simulink model "matlab_model"  (R2023a)
settings: Solver=VariableStepAuto  StartTime=0.0  StopTime=40  RelTol=1e-3
values from neighbouring files (symbols this model uses):
  contact =     [param_cina_pitch.mat]    (also in param_cina_roll.mat; param_cina_yaw.mat; verifikasi_simulasi.mat)
  control =     [param_cina_pitch.mat]    (also in param_cina_roll.mat; param_cina_yaw.mat; verifikasi_simulasi.mat)
  D = 0    [23_3_24.mat]    (also in latihanMPC.m; modelYawSpeed.mat; mpc1.mat; nonLinear.m)
  dragCoeffMov = 0.01    [23_3_24.mat]    (also in mpcDoang.mat; param_cina_pitch.mat; param_cina_roll.mat; param_cina_yaw.mat)
  dx = [dx1;dx2;dx3;dx4;dx5;dx6]    [nonLinear.m]
  g = 9.81    [param_cina_pitch.mat]    (also in param_cina_roll.mat; param_cina_yaw.mat; verifikasi_simulasi.mat)
  mass = 0.8    [nonLinear.m]    (also in param_cina_pitch.mat = 1.371; param_cina_roll.mat = 1.371; param_cina_yaw.mat = 1.371; verifikasi_simulasi.mat = 1.371)
  ModelParam_rotorCm = 8e-08    [param_cina_pitch.mat]    (also in param_cina_roll.mat; param_cina_yaw.mat)
  ModelParam_rotorCt = 4.27e-06    [param_cina_pitch.mat]    (also in param_cina_roll.mat; param_cina_yaw.mat)
  ModelParam_uavR = 0.225    [param_cina_pitch.mat]    (also in param_cina_roll.mat; param_cina_yaw.mat)
  p = angRate.Data(:,1)    [log_analisis.m]
  pitch = ATT(:,6)    [log_analisis.m]    (also in param_cina_pitch.mat = [0 0 0 0 0 0 0 0 0 0 0 0 ... (161 elements, 161x1)]; param_cina_roll.mat = [0 0 0 0 0 0 0 0 0 0 0 0 ... (161 elements, 161x1)]; param_cina_yaw.mat = [0 0 0 0 0 0 0 0 0 0 0 0 ... (161 elements, 161x1)]; verifikasi_simulasi.mat = [0 0 0 0 0 0 0 0 0 0 0 0 ... (161 elements, 161x1)])
  q = angRate.Data(:,2)    [log_analisis.m]
  r = [0 0 0 ... (first row only)    [latihanMPC.m]    (also in log_analisis.m = angRate.Data(:,3))
  ref_height = 488    [param_cina_pitch.mat]    (also in param_cina_roll.mat; param_cina_yaw.mat; verifikasi_simulasi.mat)
  ref_lat = 47.397742    [param_cina_pitch.mat]    (also in param_cina_roll.mat; param_cina_yaw.mat; verifikasi_simulasi.mat)
  ref_lon = 8.545594    [param_cina_pitch.mat]    (also in param_cina_roll.mat; param_cina_yaw.mat; verifikasi_simulasi.mat)
  roll = ATT(:,4)    [log_analisis.m]    (also in param_cina_pitch.mat = [0 0 0 0 0 0 0 0 0 0 0 0 ... (161 elements, 161x1)]; param_cina_roll.mat = [0 0 0 0 0 0 0 0 0 0 0 0 ... (161 elements, 161x1)]; param_cina_yaw.mat = [0 0 0 0 0 0 0 0 0 0 0 0 ... (161 elements, 161x1)]; verifikasi_simulasi.mat = [0 0 0 0 0 0 0 0 0 0 0 0 ... (161 elements, 161x1)])
  rotorDir = [-1 -1 1 1]    [param_cina_pitch.mat]    (also in param_cina_roll.mat; param_cina_yaw.mat; verifikasi_simulasi.mat)
  rotorPositions = [0.1815  -0.1815  0.1815  -0.1815; 0.1815  -0.1815  -0.1815  0.1815; 0  0  0  0]    [param_cina_pitch.mat]    (also in param_cina_roll.mat; param_cina_yaw.mat; verifikasi_simulasi.mat)
  rotorThrustMax = 2    [param_cina_pitch.mat]    (also in param_cina_roll.mat = 3.5; param_cina_yaw.mat = 4; verifikasi_simulasi.mat = 1.83)
  rotorTimeConst = 0.005    [param_cina_pitch.mat]    (also in param_cina_roll.mat; param_cina_yaw.mat; verifikasi_simulasi.mat)
  rotorTorqueMax = 0.06    [param_cina_pitch.mat]    (also in param_cina_roll.mat; param_cina_yaw.mat; verifikasi_simulasi.mat)
  windVel = [0 0 0]    [param_cina_pitch.mat]    (also in param_cina_roll.mat; param_cina_yaw.mat; verifikasi_simulasi.mat)
  yaw = ATT(:,8)    [log_analisis.m]    (also in param_cina_pitch.mat = [0 0 0 0 0 0 0 0 0 0 0 0 ... (161 elements, 161x1)]; param_cina_roll.mat = [0 0 0 0 0 0 0 0 0 0 0 0 ... (161 elements, 161x1)]; param_cina_yaw.mat = [0 0 0 0 0 0 0 0 0 0 0 0 ... (161 elements, 161x1)]; verifikasi_simulasi.mat = [0 0 0 0 0 0 0 0 0 0 0 0 ... (161 elements, 161x1)])
undefined symbols (not defined in the file or in its folder): ddx, ddy, ddz, dy, dz, X, Y, Z
libraries: shared6dof x1, robotcorelib x1, simulink x1, sensorgpslib x1, mspsensorlib x1
settings Model: Creator=LENOVO  LastModifiedBy=LENOVO

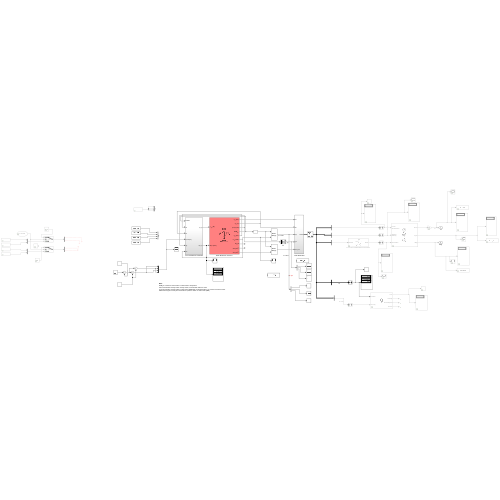
[thumbnail: Simulink's stored preview of the top-level diagram]
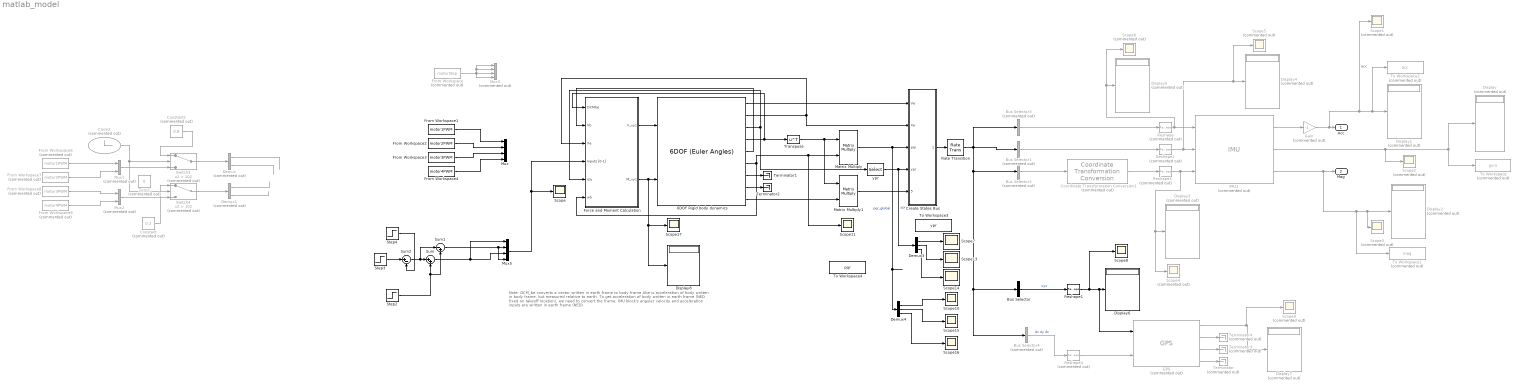
== system matlab_model ==
  note: Note:
      | DCM_be converts a vector written in earth frame to body frame
      | Abe is acceleration of body written in body frame, but measured relative to earth.
      | To get acceleration of body written in earth frame (NED fixed on takeoff location), we need to convert the frame.
      | IMU block's angular velocity and acceleration inputs are written in earth frame (NED)
  "6DOF Rigid body dynamics " : shared6dof/6DOF (Euler Angles)  units=Metric (MKS)  mtype=Fixed  rep=Quaternion  xme_0=[0,0,0]  Vm_0=init.vb  eul_0=[0;0;0]  pm_0=init.angRates  mass_0=mass  mass_e=0.5  mass_f=2.0  inertia=inertia  inertia_e=eye(3)  inertia_f=2*eye(3)  k_quat=1  vre_flag=on  abi_flag=on  aMode=aMode  xme_statename=''  Vm_statename=''  eul_statename=''  quat_statename=''  pm_statename=''  mass_statename=''
  Bus Selector : BusSelector  OutputSignals=X,Y,Z  OutputAsBus=on
  Bus Selector1 : BusSelector  Commented=on  OutputSignals=p,q,r  OutputAsBus=on
  Bus Selector2 : BusSelector  Commented=on  OutputSignals=yaw,pitch,roll  OutputAsBus=on
  Bus Selector3 : BusSelector  Commented=on  OutputSignals=ddx,ddy,ddz  OutputAsBus=on
  Bus Selector4 : BusSelector  Commented=on  OutputSignals=dx,dy,dz  OutputAsBus=on
  Clock2 : Clock  Commented=on
  Constant : Constant  Commented=on  Value=0.2
  Constant1 : Constant  Commented=on  Value=0.8
  Coordinate Transformation Conversion1 : robotcorelib/Coordinate Transformation Conversion  Commented=on  InputRepresentation=Euler Angles  InputEulerSequence=ZYX  ShowTrVecInputPort=on  OutputRepresentation=Quaternion  OutputEulerSequence=ZYX  ShowTrVecOutputPort=on  SimulateUsing=Interpreted execution
  Create States Bus : Subsystem
  Demux : Demux  Commented=on  Outputs=2
  Demux1 : Demux  Commented=on  Outputs=2
  Demux3 : Demux  Outputs=3
  Demux4 : Demux  Outputs=3
  Display{,1..5,7} (7 alike) : Display  Commented=on
  Display6 : Display
  Display8 : Display
  Force and Moment Calculation : Subsystem
  From Workspace : FromWorkspace  Commented=on  VariableName=motorStep
  From Workspace1 : FromWorkspace  VariableName=motor1PWM  SampleTime=0.25
  From Workspace2 : FromWorkspace  VariableName=motor2PWM  SampleTime=0.25
  From Workspace3 : FromWorkspace  VariableName=motor3PWM  SampleTime=0.25
  From Workspace4 : FromWorkspace  VariableName=motor4PWM  SampleTime=0.25
  From Workspace6 : FromWorkspace  Commented=on  VariableName=motor1PWM  SampleTime=0.01
  From Workspace7 : FromWorkspace  Commented=on  VariableName=motor2PWM  SampleTime=0.01
  From Workspace8 : FromWorkspace  Commented=on  VariableName=motor3PWM  SampleTime=0.01
  From Workspace9 : FromWorkspace  Commented=on  VariableName=motor4PWM  SampleTime=0.01
  GPS : sensorgpslib/GPS  Commented=on  DispRefFrame=NED  PositionInputFormat=Local  ReferenceLocation=[ref_lat ref_lon ref_height]  HorizontalPositionAccuracy=0.01  VerticalPositionAccuracy=0.01  VelocityAccuracy=0.01  DecayFactor=0.99  SeedDouble=67  SimulateUsing=Interpreted execution
      settings: LibrarySourceBlock=mspsensorlib/GPS
  Gain : Gain  Commented=on  Gain=-1
  IMU1 : mspsensorlib/IMU  Commented=on  DispRefFrame=NED  Temperature=25  MagneticFieldNED=[21.5 1.16 43.1]  MagneticFieldENU=[ -2.4169, 27.5550, 16.0849 ]  SeedDouble=87254  SimulateUsing=Interpreted execution  AccelParamsMeasurementRange=Inf  AccelParamsResolution=0  AccelParamsConstantBias=[ 0, 0, 0 ]  AccelParamsAxesMisalignment=[ 0, 0, 0 ]  AccelParamsNoiseDensity=0.0003  AccelParamsBiasInstability=[ 0, 0, 0 ]  AccelParamsRandomWalk=[ 0, 0, 0 ]  AccelParamsTemperatureBias=[ 0, 0, 0 ]  AccelParamsTemperatureScaleFactor=[ 0, 0, 0 ]  GyroParamsMeasurementRange=Inf  GyroParamsResolution=0  GyroParamsConstantBias=[ 0, 0, 0 ]  GyroParamsAxesMisalignment=[ 0, 0, 0 ]  GyroParamsAccelerationBias=0.0001  GyroParamsNoiseDensity=0.01  GyroParamsBiasInstability=[ 0, 0, 0 ]  GyroParamsRandomWalk=[ 0, 0, 0 ]  GyroParamsTemperatureBias=[ 0, 0, 0 ]  GyroParamsTemperatureScaleFactor=[ 0, 0, 0 ]  MagParamsMeasurementRange=Inf  MagParamsResolution=0  MagParamsConstantBias=[ 0, 0, 0 ]  MagParamsAxesMisalignment=[ 0, 0, 0 ]  MagParamsNoiseDensity=0.0005  MagParamsBiasInstability=[ 0, 0, 0 ]  MagParamsRandomWalk=[ 0, 0, 0 ]  MagParamsTemperatureBias=[ 0, 0, 0 ]  MagParamsTemperatureScaleFactor=[ 0, 0, 0 ]
  Matrix Multiply : Product  Multiplication=Matrix(*)
  Matrix Multiply1 : Product  Multiplication=Matrix(*)
  Mux : Mux
  Mux1 : Mux  Commented=on  Inputs=2
  Mux2 : Mux  Commented=on  Inputs=2
  Mux3 : Mux  Commented=on
  Mux5 : Mux
  Rate Transition : RateTransition  OutPortSampleTime=0.01
  Reshape{,2..4} (4 alike) : Reshape  Commented=on  OutputDimensionality=Row vector (2-D)
  Reshape1 : Reshape  OutputDimensionality=Row vector (2-D)
  Scope{,7..8,10..11,13..17} (10 alike) : Scope
  Scope{1..6,9} (7 alike) : Scope  Commented=on
  Step2 : Step  Time=0  After=0.9  SampleTime=0.25
  Step3 : Step  Time=10  After=0.01  SampleTime=0.25
  Step4 : Step  Time=11  After=0.01  SampleTime=0.25
  Sum : Sum  Inputs=|++
  Sum1 : Sum  Inputs=|-+
  Sum2 : Sum  Inputs=|+-
  Switch3 : Switch  Commented=on  Criteria=u2 > Threshold  Threshold=102  SaturateOnIntegerOverflow=off  InputSameDT=off
  Switch4 : Switch  Commented=on  Criteria=u2 > Threshold  Threshold=102  SaturateOnIntegerOverflow=off  InputSameDT=off
  Terminator : Terminator  Commented=on
  Terminator1 : Terminator
  Terminator2 : Terminator
  Terminator3 : Terminator  Commented=on
  Terminator4 : Terminator  Commented=on
  To Workspace : ToWorkspace  Commented=on  VariableName=gyro  SaveFormat=Timeseries  SampleTime=0.25
  To Workspace1 : ToWorkspace  Commented=on  VariableName=mag  SaveFormat=Timeseries  SampleTime=0.25
  To Workspace2 : ToWorkspace  Commented=on  VariableName=acc  SaveFormat=Timeseries  SampleTime=0.25
  To Workspace3 : ToWorkspace  VariableName=ypr  SaveFormat=Timeseries  SampleTime=0.25
  To Workspace4 : ToWorkspace  VariableName=pqr  SaveFormat=Timeseries  SampleTime=0.25
  Transpose : Math  Operator=transpose
  Zero1 : Constant  Commented=on  Value=0  OutDataTypeStr=Inherit: Inherit via back propagation
  ypr : Selector  InputPortWidth=3  IndexOptions=Index vector (dialog)  Indices=[3 2 1]  OutputSizes=1
  Acc : Outport
  Mag : Outport  Port=2
  wires:
  Force and Moment Calculation/2(M_xyz) -> Display8/1, Scope17/1, "6DOF Rigid body dynamics "/2
  Matrix Multiply/1 -> Demux4/1, Create States Bus/3(pqr)  "pqr_global"
  "6DOF Rigid body dynamics "/4 -> Force and Moment Calculation/1(DCMbe), Transpose/1
  "6DOF Rigid body dynamics "/3 -> Force and Moment Calculation/5(rpy), ypr/1
  "6DOF Rigid body dynamics "/5 -> Force and Moment Calculation/2(Vb)
  "6DOF Rigid body dynamics "/8 -> Terminator2/1
  "6DOF Rigid body dynamics "/7 -> Terminator1/1
  Transpose/1 -> Matrix Multiply1/1, Matrix Multiply/1
  ypr/1 -> Demux3/1, Create States Bus/4(ypr)  "ypr"
  "6DOF Rigid body dynamics "/9 -> Matrix Multiply1/2
  Force and Moment Calculation/1(F_xyz) -> "6DOF Rigid body dynamics "/1
  "6DOF Rigid body dynamics "/6 -> Scope11/1, Matrix Multiply/2, Force and Moment Calculation/6(wb)
  "6DOF Rigid body dynamics "/2 -> Create States Bus/2(Xe), Force and Moment Calculation/3(Xe)
  IMU1/2 -> Scope2/1, To Workspace/1, Display/1
  Gain/1 -> Scope1/1, To Workspace2/1, Display1/1, Acc/1  "acc"
  Reshape2/1 -> Scope5/1, Display4/1, IMU1/2
  Bus Selector2/1 -> Coordinate Transformation Conversion1/1
  Coordinate Transformation Conversion1/1 -> Reshape3/1
  Bus Selector1/1 -> Reshape2/1
  IMU1/3 -> To Workspace1/1, Scope3/1, Display2/1, Mag/1
  IMU1/1 -> Gain/1
  Bus Selector3/1 -> Reshape/1
  Reshape3/1 -> Scope4/1, Display3/1, IMU1/3
  "6DOF Rigid body dynamics "/1 -> Create States Bus/1(Ve)
  Matrix Multiply1/1 -> Create States Bus/5(acc_lnav)
  Create States Bus/1(States) -> Rate Transition/1
  Reshape/1 -> Scope6/1, Display5/1, IMU1/1
  Rate Transition/1 -> Bus Selector2/1, Bus Selector/1, Bus Selector4/1, Bus Selector1/1, Bus Selector3/1
  Bus Selector/1 -> Reshape1/1  "xyz"
  From Workspace6/1 -> Mux1/1
  From Workspace7/1 -> Mux1/2
  From Workspace8/1 -> Mux2/1
  From Workspace9/1 -> Mux2/2
  Mux1/1 -> Switch3/3
  Clock2/1 -> Switch4/2, Switch3/2
  Mux2/1 -> Switch4/3
  Switch3/1 -> Demux/1
  Switch4/1 -> Demux1/1
  Demux1/1 -> ?
  Demux1/2 -> ?
  Demux/1 -> ?
  Demux/2 -> ?
  Reshape1/1 -> Scope8/1, GPS/1, Display6/1
  Bus Selector4/1 -> Reshape4/1  "dx dy dz"
  Reshape4/1 -> GPS/2
  GPS/4 -> Terminator/1
  GPS/3 -> Terminator3/1
  GPS/2 -> Terminator4/1
  GPS/1 -> Scope9/1, Display7/1
  Constant/1 -> Switch4/1
  Constant1/1 -> Switch3/1
  From Workspace1/1 -> Mux/1
  From Workspace2/1 -> Mux/2
  From Workspace3/1 -> Mux/3
  From Workspace4/1 -> Mux/4
  From Workspace/1 -> Mux3/1, Mux3/2, Mux3/4, Mux3/3
  Demux3/2 -> Scope13/1
  Demux3/3 -> Scope14/1
  Demux3/1 -> Scope7/1
  Demux4/1 -> Scope10/1
  Demux4/2 -> Scope15/1
  Demux4/3 -> Scope16/1
  Step3/1 -> Sum2/1
  Sum1/1 -> Mux5/4, Mux5/2
  Step2/1 -> Sum1/2, Sum/2
  Sum2/1 -> Sum1/1, Sum/1
  Sum/1 -> Mux5/1, Mux5/3
  Step4/1 -> Sum2/2
  Mux5/1 -> Force and Moment Calculation/4(Inputs [0-1]), Scope/1

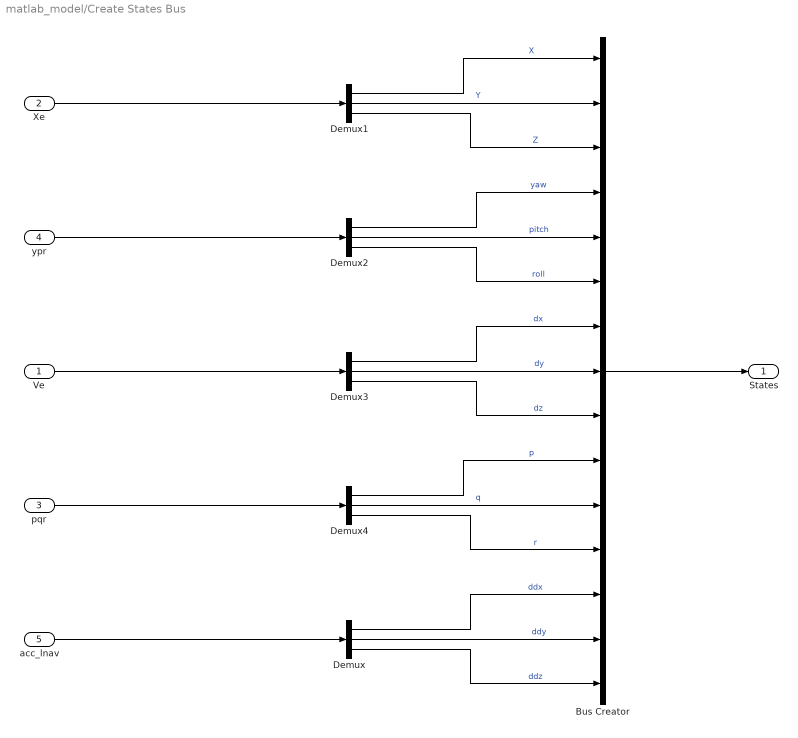
== system matlab_model/Create States Bus ==
  Ve : Inport
  Xe : Inport  Port=2
  pqr : Inport  Port=3
  ypr : Inport  Port=4
  acc_lnav : Inport  Port=5
  Bus Creator : BusCreator  Inputs=X,Y,Z,yaw,pitch,roll,dx,dy,dz,p,q,r,ddx,ddy,ddz
  Demux{,1..4} (5 alike) : Demux  Outputs=3
  States : Outport
  wires:
  Demux1/1 -> Bus Creator/1  "X"
  Demux1/2 -> Bus Creator/2  "Y"
  ypr/1 -> Demux2/1
  Demux2/2 -> Bus Creator/5  "pitch"
  Demux3/2 -> Bus Creator/8  "dy"
  Demux2/3 -> Bus Creator/6  "roll"
  pqr/1 -> Demux4/1
  Ve/1 -> Demux3/1
  Demux2/1 -> Bus Creator/4  "yaw"
  Demux1/3 -> Bus Creator/3  "Z"
  Demux3/1 -> Bus Creator/7  "dx"
  Demux4/2 -> Bus Creator/11  "q"
  Demux3/3 -> Bus Creator/9  "dz"
  Demux4/3 -> Bus Creator/12  "r"
  Demux4/1 -> Bus Creator/10  "p"
  Bus Creator/1 -> States/1
  Xe/1 -> Demux1/1
  acc_lnav/1 -> Demux/1
  Demux/3 -> Bus Creator/15  "ddz"
  Demux/2 -> Bus Creator/14  "ddy"
  Demux/1 -> Bus Creator/13  "ddx"

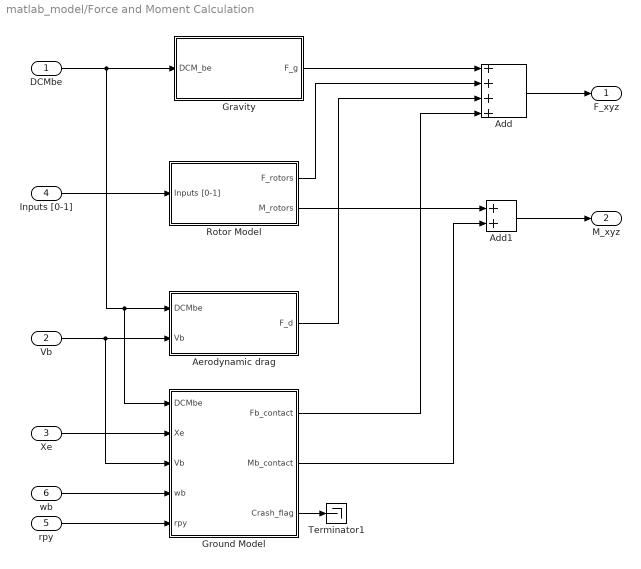
== system matlab_model/Force and Moment Calculation ==
  DCMbe : Inport
  Vb : Inport  Port=2
  Xe : Inport  Port=3
  Inputs [0-1] : Inport  Port=4
  rpy : Inport  Port=5
  wb : Inport  Port=6
  Add : Sum  Inputs=++++
  Add1 : Sum
  Aerodynamic drag : Subsystem
  Gravity : Subsystem
  Ground Model : Subsystem
  Rotor Model : Subsystem
  Terminator1 : Terminator
  F_xyz : Outport
  M_xyz : Outport  Port=2
  wires:
  Inputs [0-1]/1 -> Rotor Model/1(Inputs [0-1])
  DCMbe/1 -> Ground Model/1(DCMbe), Aerodynamic drag/1(DCMbe), Gravity/1(DCM_be)
  Gravity/1(F_g) -> Add/1
  Add/1 -> F_xyz/1
  Vb/1 -> Ground Model/3(Vb), Aerodynamic drag/2(Vb)
  Rotor Model/1(F_rotors) -> Add/2
  Aerodynamic drag/1(F_d) -> Add/3
  Xe/1 -> Ground Model/2(Xe)
  wb/1 -> Ground Model/4(wb)
  rpy/1 -> Ground Model/5(rpy)
  Rotor Model/2(M_rotors) -> Add1/1
  Ground Model/2(Mb_contact) -> Add1/2
  Add1/1 -> M_xyz/1
  Ground Model/1(Fb_contact) -> Add/4
  Ground Model/3(Crash_flag) -> Terminator1/1

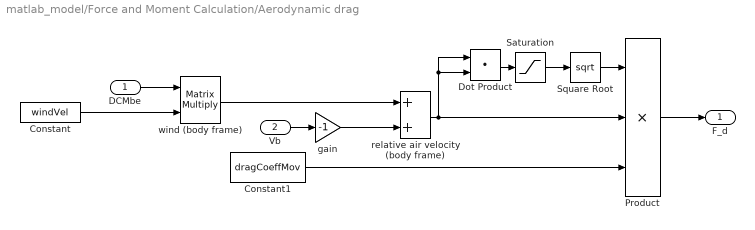
== system matlab_model/Force and Moment Calculation/Aerodynamic drag ==
  DCMbe : Inport
  Vb : Inport  Port=2
  Constant : Constant  Value=windVel
  Constant1 : Constant  Value=dragCoeffMov
  Dot Product : DotProduct  OutDataTypeStr=Inherit: Inherit via internal rule
  Product : Product  Inputs=3
  Saturation : Saturate  UpperLimit=inf  LowerLimit=0.0001
  Square Root : Sqrt
  gain : Gain  Gain=-1
  relative air velocity (body frame) : Sum
  wind (body frame) : Product  Multiplication=Matrix(*)
  F_d : Outport
  wires:
  relative air velocity (body frame)/1 -> Dot Product/2, Dot Product/1, Product/2
  DCMbe/1 -> wind (body frame)/1
  Product/1 -> F_d/1
  Saturation/1 -> Square Root/1
  Vb/1 -> gain/1
  Dot Product/1 -> Saturation/1
  Square Root/1 -> Product/1
  wind (body frame)/1 -> relative air velocity (body frame)/1
  gain/1 -> relative air velocity (body frame)/2
  Constant1/1 -> Product/3
  Constant/1 -> wind (body frame)/2

== system matlab_model/Force and Moment Calculation/Gravity ==
  DCM_be : Inport
  Constant : Constant  Value=[0 0 g]'
  Gain : Gain  Gain=mass
  Matrix Multiply : Product  Multiplication=Matrix(*)
  F_g : Outport
  wires:
  Matrix Multiply/1 -> Gain/1
  Constant/1 -> Matrix Multiply/2
  DCM_be/1 -> Matrix Multiply/1
  Gain/1 -> F_g/1

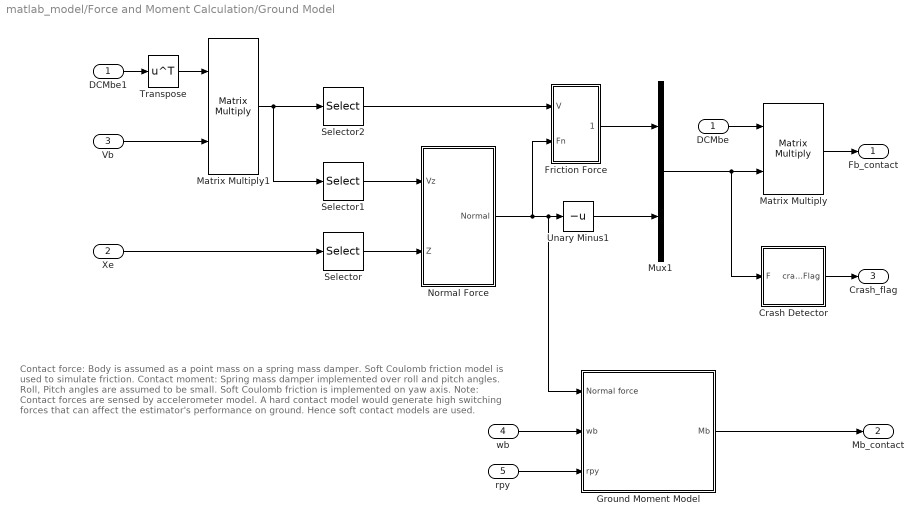
== system matlab_model/Force and Moment Calculation/Ground Model ==
  note: Contact force:
      | Body is assumed as a point mass on a spring mass damper. Soft Coulomb friction model is used to simulate friction.
      |
      | Contact moment:
      | Spring mass damper implemented over roll and pitch angles. Roll, Pitch angles are assumed to be small.
      | Soft Coulomb friction is implemented on yaw axis.
      |
      | Note:
      | Contact forces are sensed by accelerometer model. A hard contact model would generate high switching forces that can affect the estimator's performance on ground. Hence soft contact models are used.
  DCMbe : Inport
  Xe : Inport  Port=2
  Vb : Inport  Port=3
  wb : Inport  Port=4
  rpy : Inport  Port=5
  Crash Detector : Subsystem
  DCMbe1 : InportShadow
  Friction Force : Subsystem
  Ground Moment Model : Subsystem
  Matrix Multiply : Product  Multiplication=Matrix(*)
  Matrix Multiply1 : Product  Multiplication=Matrix(*)
  Mux1 : Mux  Inputs=2
  Normal Force : Subsystem
  Selector : Selector  InputPortWidth=3  IndexOptions=Index vector (dialog)  Indices=[3]  OutputSizes=1
  Selector1 : Selector  InputPortWidth=3  IndexOptions=Index vector (dialog)  Indices=[3]  OutputSizes=1
  Selector2 : Selector  InputPortWidth=3  IndexOptions=Index vector (dialog)  Indices=[1,2]  OutputSizes=1
  Transpose : Math  Operator=transpose
  Unary Minus1 : UnaryMinus
  Fb_contact : Outport
  Mb_contact : Outport  Port=2
  Crash_flag : Outport  Port=3
  wires:
  Crash Detector/1(crashFlag) -> Crash_flag/1
  Xe/1 -> Selector/1
  Selector1/1 -> Normal Force/1(Vz)
  Selector/1 -> Normal Force/2(Z)
  DCMbe/1 -> Matrix Multiply/1
  Matrix Multiply/1 -> Fb_contact/1
  Normal Force/1(Normal) -> Ground Moment Model/1(Normal force), Unary Minus1/1, Friction Force/2(Fn)
  Mux1/1 -> Crash Detector/1(F), Matrix Multiply/2
  Unary Minus1/1 -> Mux1/2
  Selector2/1 -> Friction Force/1(V)
  Friction Force/1(Friction) -> Mux1/1
  DCMbe1/1 -> Transpose/1
  Transpose/1 -> Matrix Multiply1/1
  Vb/1 -> Matrix Multiply1/2
  Matrix Multiply1/1 -> Selector1/1, Selector2/1
  wb/1 -> Ground Moment Model/2(wb)
  rpy/1 -> Ground Moment Model/3(rpy)
  Ground Moment Model/1(Mb) -> Mb_contact/1

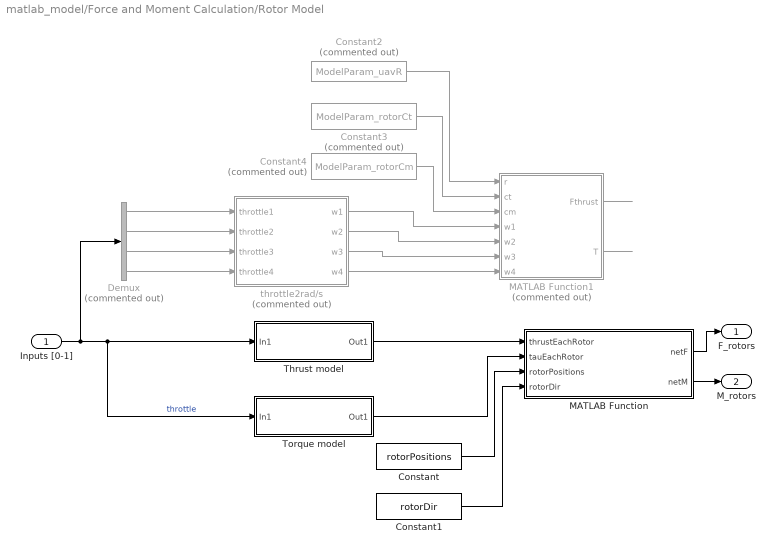
== system matlab_model/Force and Moment Calculation/Rotor Model ==
  Inputs [0-1] : Inport
  Constant : Constant  Value=rotorPositions
  Constant1 : Constant  Value=rotorDir
  Constant2 : Constant  Commented=on  Value=ModelParam_uavR
  Constant3 : Constant  Commented=on  Value=ModelParam_rotorCt
  Constant4 : Constant  Commented=on  Value=ModelParam_rotorCm
  Demux : Demux  Commented=on
  MATLAB Function : MATLAB Function  TreatAsAtomicUnit=on
  MATLAB Function1 : MATLAB Function  Commented=on  TreatAsAtomicUnit=on
  Thrust model : Subsystem
  Torque model : Subsystem
  throttle2rad/s : Subsystem  Commented=on
  F_rotors : Outport
  M_rotors : Outport  Port=2
  wires:
  Inputs [0-1]/1 -> Torque model/1(In1), Thrust model/1(In1), Demux/1  "throttle"
  MATLAB Function/1(netF) -> F_rotors/1
  MATLAB Function/2(netM) -> M_rotors/1
  Constant/1 -> MATLAB Function/3(rotorPositions)
  Constant1/1 -> MATLAB Function/4(rotorDir)
  Torque model/1(Out1) -> MATLAB Function/2(tauEachRotor)
  Thrust model/1(Out1) -> MATLAB Function/1(thrustEachRotor)
  throttle2rad/s/1(w1) -> MATLAB Function1/4(w1)
  throttle2rad/s/2(w2) -> MATLAB Function1/5(w2)
  throttle2rad/s/3(w3) -> MATLAB Function1/6(w3)
  throttle2rad/s/4(w4) -> MATLAB Function1/7(w4)
  Demux/4 -> throttle2rad/s/4(throttle4)
  Demux/3 -> throttle2rad/s/3(throttle3)
  Demux/2 -> throttle2rad/s/2(throttle2)
  Demux/1 -> throttle2rad/s/1(throttle1)
  Constant2/1 -> MATLAB Function1/1(r)
  MATLAB Function1/2(T) -> ?
  MATLAB Function1/1(Fthrust) -> ?
  Constant3/1 -> MATLAB Function1/2(ct)
  Constant4/1 -> MATLAB Function1/3(cm)

== system matlab_model/Force and Moment Calculation/Ground Model/Crash Detector ==
  F : Inport
  Compare To Constant : simulink/Logic and Bit Operations/Compare To Constant  relop=>  const=100  OutDataTypeStr=boolean
  Gain : Gain  Gain=1/mass/g
  norm1 : Subsystem
  crashFlag : Outport
  wires:
  F/1 -> norm1/1(F)
  norm1/1(Out1) -> Gain/1
  Compare To Constant/1 -> crashFlag/1
  Gain/1 -> Compare To Constant/1  "g's"

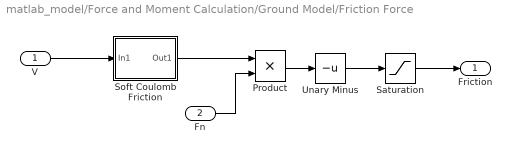
== system matlab_model/Force and Moment Calculation/Ground Model/Friction Force ==
  V : Inport
  Fn : Inport  Port=2
  Product : Product
  Saturation : Saturate  UpperLimit=contact.translation.maxFriction  LowerLimit=-contact.translation.maxFriction
  Soft Coulomb Friction : Subsystem
  Unary Minus : UnaryMinus
  Friction : Outport
  wires:
  Fn/1 -> Product/2
  Soft Coulomb Friction/1(Out1) -> Product/1
  Product/1 -> Unary Minus/1
  V/1 -> Soft Coulomb Friction/1(In1)
  Unary Minus/1 -> Saturation/1
  Saturation/1 -> Friction/1

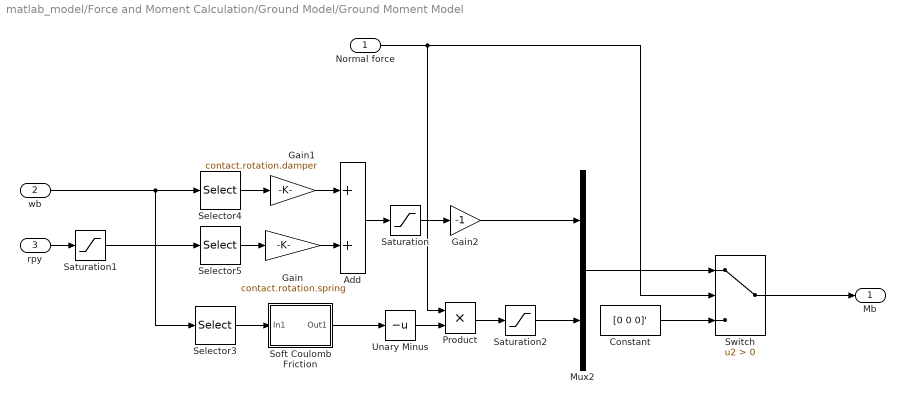
== system matlab_model/Force and Moment Calculation/Ground Model/Ground Moment Model ==
  Normal force : Inport
  wb : Inport  Port=2
  rpy : Inport  Port=3
  Add : Sum
  Constant : Constant  Value=[0 0 0]'
  Gain : Gain  Gain=contact.rotation.spring
  Gain1 : Gain  Gain=contact.rotation.damper
  Gain2 : Gain  Gain=-1
  Mux2 : Mux  Inputs=2
  Product : Product
  Saturation : Saturate  UpperLimit=control.rotation.maxMoment  LowerLimit=-control.rotation.maxMoment
  Saturation1 : Saturate  UpperLimit=20*pi/180  LowerLimit=-20*pi/180
  Saturation2 : Saturate  UpperLimit=control.rotation.maxMoment  LowerLimit=-control.rotation.maxMoment
  Selector3 : Selector  InputPortWidth=3  IndexOptions=Index vector (dialog)  Indices=[3]  OutputSizes=1
  Selector4 : Selector  InputPortWidth=3  IndexOptions=Index vector (dialog)  Indices=[1, 2]  OutputSizes=1
  Selector5 : Selector  InputPortWidth=3  IndexOptions=Index vector (dialog)  Indices=[1, 2]  OutputSizes=1
  Soft Coulomb Friction : Subsystem
  Switch : Switch  Criteria=u2 > Threshold  SaturateOnIntegerOverflow=off  InputSameDT=off
  Unary Minus : UnaryMinus
  Mb : Outport
  wires:
  Gain2/1 -> Mux2/1
  Add/1 -> Saturation/1
  Gain/1 -> Add/2
  Saturation/1 -> Gain2/1
  Selector4/1 -> Gain1/1
  Gain1/1 -> Add/1
  Constant/1 -> Switch/3
  Selector5/1 -> Gain/1
  Switch/1 -> Mb/1
  Mux2/1 -> Switch/1
  Normal force/1 -> Product/1, Switch/2
  rpy/1 -> Saturation1/1
  Saturation1/1 -> Selector5/1
  wb/1 -> Selector4/1, Selector3/1
  Selector3/1 -> Soft Coulomb Friction/1(In1)
  Soft Coulomb Friction/1(Out1) -> Unary Minus/1
  Unary Minus/1 -> Product/2
  Product/1 -> Saturation2/1
  Saturation2/1 -> Mux2/2

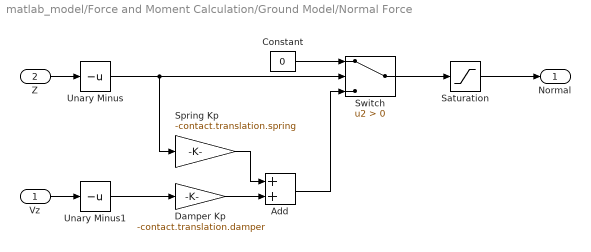
== system matlab_model/Force and Moment Calculation/Ground Model/Normal Force ==
  Vz : Inport
  Z : Inport  Port=2
  Add : Sum
  Constant : Constant  Value=0
  Damper Kp : Gain  Gain=-contact.translation.damper
  Saturation : Saturate  UpperLimit=contact.translation.maxNormal  LowerLimit=0
  Spring Kp : Gain  Gain=-contact.translation.spring
  Switch : Switch  Criteria=u2 > Threshold  SaturateOnIntegerOverflow=off  InputSameDT=off
  Unary Minus : UnaryMinus
  Unary Minus1 : UnaryMinus
  Normal : Outport
  wires:
  Constant/1 -> Switch/1
  Z/1 -> Unary Minus/1
  Switch/1 -> Saturation/1
  Damper Kp/1 -> Add/2
  Add/1 -> Switch/3
  Spring Kp/1 -> Add/1
  Vz/1 -> Unary Minus1/1
  Saturation/1 -> Normal/1
  Unary Minus/1 -> Spring Kp/1, Switch/2
  Unary Minus1/1 -> Damper Kp/1

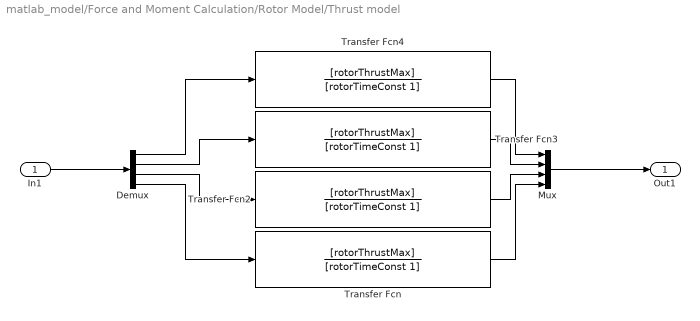
== system matlab_model/Force and Moment Calculation/Rotor Model/Thrust model ==
  In1 : Inport
  Demux : Demux
  Mux : Mux
  Transfer Fcn{,2..4} (4 alike) : TransferFcn  Numerator=[rotorThrustMax]  Denominator=[rotorTimeConst 1]
  Out1 : Outport
  wires:
  Transfer Fcn3/1 -> Mux/2
  Demux/1 -> Transfer Fcn4/1
  Transfer Fcn2/1 -> Mux/3
  Demux/3 -> Transfer Fcn2/1
  Mux/1 -> Out1/1
  Transfer Fcn4/1 -> Mux/1
  Demux/4 -> Transfer Fcn/1
  Demux/2 -> Transfer Fcn3/1
  Transfer Fcn/1 -> Mux/4
  In1/1 -> Demux/1

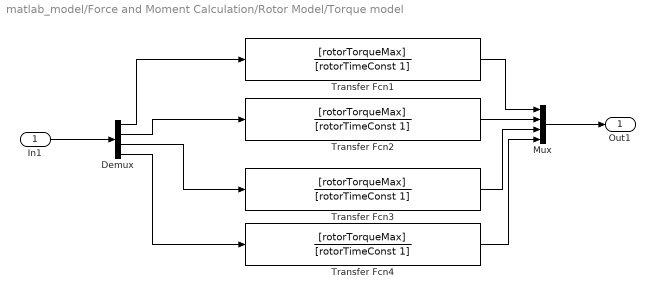
== system matlab_model/Force and Moment Calculation/Rotor Model/Torque model ==
  In1 : Inport
  Demux : Demux
  Mux : Mux
  Transfer Fcn{1..4} (4 alike) : TransferFcn  Numerator=[rotorTorqueMax]  Denominator=[rotorTimeConst 1]
  Out1 : Outport
  wires:
  Transfer Fcn4/1 -> Mux/4
  Demux/1 -> Transfer Fcn1/1
  Transfer Fcn3/1 -> Mux/3
  Transfer Fcn2/1 -> Mux/2
  Demux/2 -> Transfer Fcn2/1
  Demux/4 -> Transfer Fcn4/1
  Demux/3 -> Transfer Fcn3/1
  Mux/1 -> Out1/1
  Transfer Fcn1/1 -> Mux/1
  In1/1 -> Demux/1

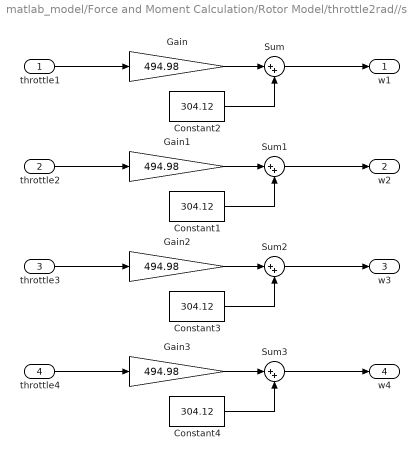
== system matlab_model/Force and Moment Calculation/Rotor Model/throttle2rad//s ==
  throttle1 : Inport
  throttle2 : Inport  Port=2
  throttle3 : Inport  Port=3
  throttle4 : Inport  Port=4
  Constant{1..4} (4 alike) : Constant  Value=304.12
  Gain{,1..3} (4 alike) : Gain  Gain=494.98
  Sum{,1..3} (4 alike) : Sum  Inputs=|++
  w1 : Outport
  w2 : Outport  Port=2
  w3 : Outport  Port=3
  w4 : Outport  Port=4
  wires:
  Gain/1 -> Sum/1
  throttle1/1 -> Gain/1
  Constant2/1 -> Sum/2
  Constant1/1 -> Sum1/2
  Gain1/1 -> Sum1/1
  throttle2/1 -> Gain1/1
  Constant3/1 -> Sum2/2
  Sum2/1 -> w3/1
  Gain2/1 -> Sum2/1
  throttle3/1 -> Gain2/1
  Constant4/1 -> Sum3/2
  Sum3/1 -> w4/1
  Gain3/1 -> Sum3/1
  throttle4/1 -> Gain3/1
  Sum1/1 -> w2/1
  Sum/1 -> w1/1

== system matlab_model/Force and Moment Calculation/Ground Model/Crash Detector/norm1 ==
  F : Inport
  Dot Product : DotProduct  OutDataTypeStr=Inherit: Inherit via internal rule
  Sqrt : Sqrt
  Out1 : Outport
  wires:
  Dot Product/1 -> Sqrt/1
  F/1 -> Dot Product/2, Dot Product/1
  Sqrt/1 -> Out1/1

== system matlab_model/Force and Moment Calculation/Ground Model/Friction Force/Soft Coulomb Friction ==
  note: Pennestrì, E., Rossi, V., Salvini, P. et al. Review and comparison of dry friction force models. Nonlinear Dyn 83, 1785–1801 (2016). https://doi.org/10.1007/s11071-015-2485-3
  In1 : Inport
  Tanh : Trigonometry  Operator=tanh
  friction coefficient : Gain  Gain=contact.translation.friction
  vd : Gain  Gain=1/contact.translation.vd
  Out1 : Outport
  wires:
  In1/1 -> vd/1
  vd/1 -> Tanh/1
  Tanh/1 -> friction coefficient/1
  friction coefficient/1 -> Out1/1

== system matlab_model/Force and Moment Calculation/Ground Model/Ground Moment Model/Soft Coulomb Friction ==
  note: Pennestrì, E., Rossi, V., Salvini, P. et al. Review and comparison of dry friction force models. Nonlinear Dyn 83, 1785–1801 (2016). https://doi.org/10.1007/s11071-015-2485-3
  In1 : Inport
  Tanh : Trigonometry  Operator=tanh
  friction coefficient : Gain  Gain=control.rotation.friction
  vd : Gain  Gain=1/control.rotation.vd
  Out1 : Outport
  wires:
  In1/1 -> vd/1
  vd/1 -> Tanh/1
  Tanh/1 -> friction coefficient/1
  friction coefficient/1 -> Out1/1

== matlab function matlab_model/Force and Moment Calculation/Rotor Model/MATLAB Function1 ==
  data: r input; ct input; cm input; w1 input; Fthrust output; T output; w2 input; w3 input; w4 input
function [Fthrust,T] = fcn(r,ct,cm,w1,w2,w3,w4)
Fthrust = [0; 0; -ct*(w1^2+w2^2+w3^2+w4^2)];
Tx = r*ct/sqrt(2)*(w1^2-w2^2-w3^2+w4^2);
Ty = r*ct/sqrt(2)*(w1^2+w2^2-w3^2-w4^2);
Tz = cm*(w1^2+w2^2+w3^2+w4^2);
T = [Tx; Ty; Tz];

== matlab function matlab_model/Force and Moment Calculation/Rotor Model/MATLAB Function ==
  data: thrustEachRotor input; tauEachRotor input; rotorPositions input; netF output; netM output; rotorDir input
function [netF, netM] = getForceMoment(thrustEachRotor, tauEachRotor, rotorPositions, rotorDir)
%#codegen
Fx = 0;
Fy = 0;
Fz = -sum(thrustEachRotor);

netF = [Fx; Fy; Fz];

netM = [0; 0; 0]; %initialize
    for i = 1:4
        rotPos = rotorPositions(:, i);
        Fi = [0, 0, -thrustEachRotor(i)]';
        netM = netM +  cross(rotPos, Fi);%contribution from thrusts of each propeller
        netM(3) = netM(3) - rotorDir(i)*tauEachRotor(i); %contribution from counter torque acting on propeller
    end

end
